simulink model "SetReset"  (Simulink 6.0)
settings: Solver=FixedStepDiscrete  StartTime=0.0  StopTime=inf  RelTol=1e-3
settings Model: Creator=scaife  LastModifiedBy=scaife  ExtModeAutoUpdateStatusClock=off
settings DataIOCC: SignalLoggingName=sigsOut
settings DebuggingCC: SolverPrmCheckMsg=none
settings HardwareCC: TargetUnknown=on
settings GRTTargetCC: ModelReferenceCompliant=off  MatFileLogging=off

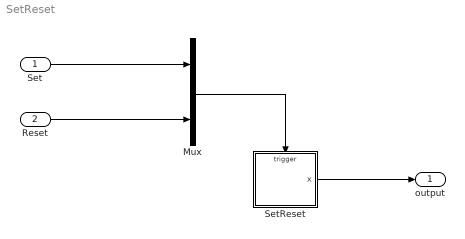
== system SetReset ==
  Set : Inport  Port=1  LatchInput=off
  Reset : Inport  Port=2  LatchInput=off
  Mux : Mux  Inputs=2
  SetReset : Stateflow chart
  output : Outport
  wires:
  Mux/1 -> SetReset/Trigger
  Set/1 -> Mux/1
  Reset/1 -> Mux/2
  SetReset/1(x) -> output/1

== stateflow chart SetReset ==
  state Off/
    en:x=0
  state On/
    en:x=1
  Off -> On : Set
  On -> Off : Reset
  (default) -> Off
  data: x output int32
  events: Set input RISING_EDGE_EVENT; Reset input RISING_EDGE_EVENT
